simulink model "tower_model"  (Simulink 7.9)
settings: Solver=VariableStepDiscrete  StartTime=0.0  StopTime=10.0  RelTol=1e-3
undefined symbols (not defined in the file or in its folder): tower, tower_x0, tower_xref, Ts
libraries: simulink x1
settings Model: Creator=matias  LastModifiedBy=matias

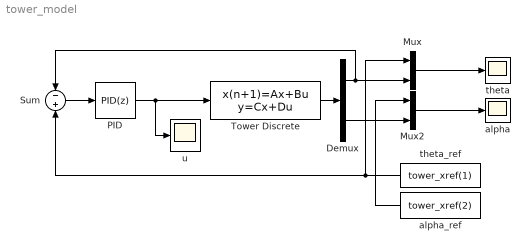
== system tower_model ==
  Demux : Demux  Outputs=2
  Mux : Mux  Inputs=2
  Mux2 : Mux  Inputs=2
  PID : simulink/Continuous/PID Controller  Controller=PID  TimeDomain=Discrete-time  SampleTime=Ts  IntegratorMethod=Forward Euler  FilterMethod=Forward Euler  Form=Parallel  P=0.01  I=0  D=0  N=100  InitialConditionSource=internal  InitialConditionForIntegrator=0  InitialConditionForFilter=0  ExternalReset=none  LimitOutput=off  UpperSaturationLimit=1  LowerSaturationLimit=-1  LinearizeAsGain=off  AntiWindupMode=clamping  Kb=1  TrackingMode=off  Kt=1  PParamMin=[]  PParamMax=[]  IParamMin=[]  IParamMax=[]  DParamMin=[]  DParamMax=[]  NParamMin=[]  NParamMax=[]  KbParamMin=[]  KbParamMax=[]  KtParamMin=[]  KtParamMax=[]  POutMin=[]  POutMax=[]  IOutMin=[]  IOutMax=[]  DOutMin=[]  DOutMax=[]  NOutMin=[]  NOutMax=[]  KbOutMin=[]  KbOutMax=[]  KtOutMin=[]  KtOutMax=[]  IntegratorOutMin=[]  IntegratorOutMax=[]  FilterOutMin=[]  FilterOutMax=[]  SumOutMin=[]  SumOutMax=[]  SumI1OutMin=[]  SumI1OutMax=[]  SumI2OutMin=[]  SumI2OutMax=[]  SumI3OutMin=[]  SumI3OutMax=[]  SumDOutMin=[]  SumDOutMax=[]  SaturationOutMin=[]  SaturationOutMax=[]  IntegratorContinuousStateAttributes=''  IntegratorStateMustResolveToSignalObject=off  IntegratorRTWStateStorageClass=Auto  FilterContinuousStateAttributes=''  FilterStateMustResolveToSignalObject=off  FilterRTWStateStorageClass=Auto
  Sum : Sum  Inputs=-|+  SampleTime=Ts
  Tower Discrete : DiscreteStateSpace  A=tower.A  B=tower.B  C=tower.C(tower.OutputGroup.MO,:)  D=tower.D(tower.OutputGroup.MO,:)  X0=tower_x0  SampleTime=Ts
  alpha : Scope
      settings: TimeRange=10
  alpha_ref : Constant  Value=tower_xref(2)
  theta : Scope
      settings: YMin=-220  YMax=10
  theta_ref : Constant  Value=tower_xref(1)
  u : Scope
      settings: YMin=-5500  YMax=6000  SaveName=ScopeData2
  wires:
  Tower Discrete/1 -> Demux/1
  Mux/1 -> theta/1
  theta_ref/1 -> Mux/1, Sum/2
  Mux2/1 -> alpha/1
  Demux/1 -> Mux/2, Sum/1
  alpha_ref/1 -> Mux2/1
  Demux/2 -> Mux2/2
  Sum/1 -> PID/1
  PID/1 -> u/1, Tower Discrete/1
